simulink model "final"  (R2023b)
settings: Solver=ode4  StartTime=0.0  StopTime=10.0  FixedStep=0.001  RelTol=1e-3
settings Model: Creator=ratho  LastModifiedBy=ratho

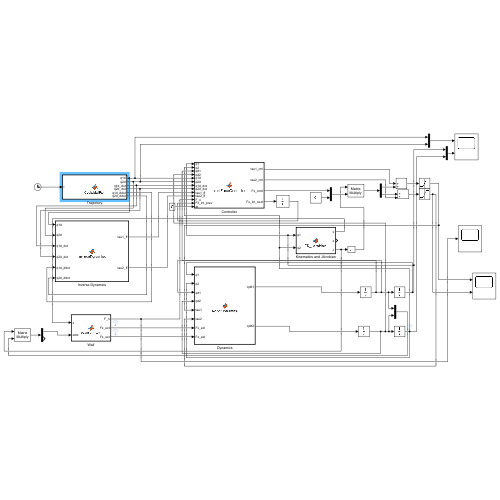
[thumbnail: Simulink's stored preview of the top-level diagram]
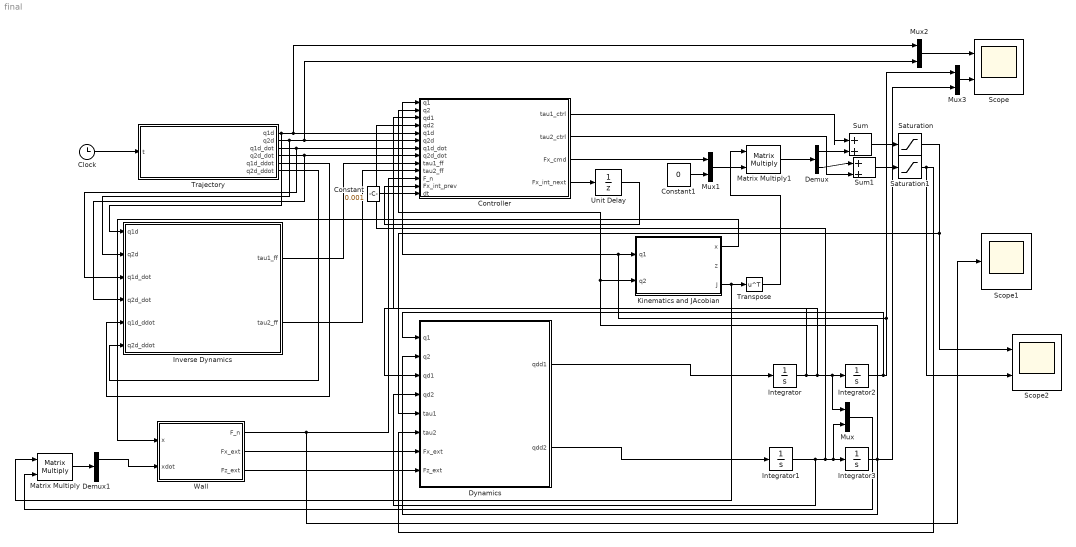
== system final ==
  Clock : Clock
  Constant : Constant  Value=0.001
  Constant1 : Constant  Value=0
  Controller : MATLAB Function  TreatAsAtomicUnit=on
  Demux : Demux  Outputs=2
  Demux1 : Demux  Outputs=2
  Dynamics : MATLAB Function  TreatAsAtomicUnit=on
  Integrator : Integrator
  Integrator1 : Integrator
  Integrator2 : Integrator  InitialCondition=pi/3
  Integrator3 : Integrator  InitialCondition=-pi/4
  Inverse Dynamics : MATLAB Function  TreatAsAtomicUnit=on
  Kinematics and JAcobian : MATLAB Function  TreatAsAtomicUnit=on
  Matrix Multiply : Product  Multiplication=Matrix(*)
  Matrix Multiply1 : Product  Multiplication=Matrix(*)
  Mux{,1..3} (4 alike) : Mux  Inputs=2
  Saturation : Saturate  UpperLimit=400  LowerLimit=-400
  Saturation1 : Saturate  UpperLimit=400  LowerLimit=-400
  Scope : Scope  NumInputPorts=2
  Scope1 : Scope
  Scope2 : Scope  NumInputPorts=2
  Sum : Sum  Inputs=|++
  Sum1 : Sum  Inputs=|++
  Trajectory : MATLAB Function  TreatAsAtomicUnit=on
  Transpose : Math  Operator=transpose
  Unit Delay : UnitDelay  SampleTime=0.001  HasFrameUpgradeWarning=on
  Wall : MATLAB Function  TreatAsAtomicUnit=on
  wires:
  Clock/1 -> Trajectory/1(t)
  Dynamics/1(qdd1) -> Integrator/1
  Dynamics/2(qdd2) -> Integrator1/1
  Integrator/1 -> Dynamics/3(qd1), Controller/3(qd1), Mux/1, Integrator2/1
  Integrator1/1 -> Dynamics/4(qd2), Controller/4(qd2), Mux/2, Integrator3/1
  Integrator2/1 -> Dynamics/1(q1), Mux3/1, Kinematics and JAcobian/1(q1), Controller/1(q1)
  Integrator3/1 -> Mux3/2, Controller/2(q2), Kinematics and JAcobian/2(q2), Dynamics/2(q2)
  Trajectory/1(q1d) -> Mux2/1, Controller/5(q1d), Inverse Dynamics/1(q1d)
  Trajectory/2(q2d) -> Mux2/2, Controller/6(q2d), Inverse Dynamics/2(q2d)
  Trajectory/3(q1d_dot) -> Controller/7(q1d_dot), Inverse Dynamics/3(q1d_dot)
  Trajectory/4(q2d_dot) -> Controller/8(q2d_dot), Inverse Dynamics/4(q2d_dot)
  Trajectory/5(q1d_ddot) -> Inverse Dynamics/5(q1d_ddot)
  Trajectory/6(q2d_ddot) -> Inverse Dynamics/6(q2d_ddot)
  Inverse Dynamics/1(tau1_ff) -> Controller/9(tau1_ff)
  Inverse Dynamics/2(tau2_ff) -> Controller/10(tau2_ff)
  Wall/2(Fx_ext) -> Dynamics/7(Fx_ext)
  Wall/3(Fz_ext) -> Dynamics/8(Fz_ext)
  Kinematics and JAcobian/1(x) -> Wall/1(x)
  Constant/1 -> Controller/13(dt)
  Controller/4(Fx_int_next) -> Unit Delay/1
  Unit Delay/1 -> Controller/12(Fx_int_prev)
  Kinematics and JAcobian/3(J) -> Matrix Multiply/1, Transpose/1
  Mux/1 -> Matrix Multiply/2
  Controller/3(Fx_cmd) -> Mux1/1
  Constant1/1 -> Mux1/2
  Mux1/1 -> Matrix Multiply1/2
  Transpose/1 -> Matrix Multiply1/1
  Matrix Multiply1/1 -> Demux/1
  Demux/2 -> Sum1/1
  Demux/1 -> Sum/2
  Controller/1(tau1_ctrl) -> Sum/1
  Controller/2(tau2_ctrl) -> Sum1/2
  Sum/1 -> Saturation/1
  Sum1/1 -> Saturation1/1
  Matrix Multiply/1 -> Demux1/1
  Demux1/1 -> Wall/2(xdot)
  Saturation/1 -> Scope2/1, Dynamics/5(tau1)
  Saturation1/1 -> Scope2/2, Dynamics/6(tau2)
  Mux2/1 -> Scope/1
  Mux3/1 -> Scope/2
  Wall/1(F_n) -> Scope1/1, Controller/11(F_n)

== matlab function final/Inverse Dynamics ==
  data: q1d input; tau1_ff output; q2d input; q1d_dot input; q2d_dot input; q1d_ddot input; q2d_ddot input; tau2_ff output
function [tau1_ff, tau2_ff] = InverseDynamics( ...
    q1d,q2d,q1d_dot,q2d_dot,q1d_ddot,q2d_ddot)
%#codegen

%% ---- CONSTANTS ----
m1 = 1; m2 = 1;
l1 = 1; l2 = 1;
r1 = l1/2; r2 = l2/2;
I1 = (1/12)*m1*l1^2;
I2 = (1/12)*m2*l2^2;
g  = 9.81;

%% ---- Inertia ----
M11 = I1+I2 + m1*r1^2 + m2*(l1^2+r2^2) + 2*m2*l1*r2*cos(q2d);
M12 = I2 + m2*r2^2 + m2*l1*r2*cos(q2d);
M21 = M12;
M22 = I2 + m2*r2^2;
M = [M11 M12; M21 M22];

%% ---- Coriolis ----
h  = -m2*l1*r2*sin(q2d);
C1 = h*(2*q1d_dot*q2d_dot + q2d_dot^2);
C2 = h*(-q1d_dot^2);
C  = [C1; C2];

%% ---- Gravity ----
G1 = (m1*r1 + m2*l1)*g*cos(q1d) + m2*r2*g*cos(q1d+q2d);
G2 = m2*r2*g*cos(q1d+q2d);
G  = [G1; G2];

tau = M*[q1d_ddot; q2d_ddot] + C + G;

tau1_ff = tau(1);
tau2_ff = tau(2);

end

== matlab function final/Wall ==
  data: x input; F_n output; xdot input; Fx_ext output; Fz_ext output
function [F_n, Fx_ext, Fz_ext] = WallContact(x, xdot)
%#codegen

% ==== CONSTANTS ====
wall_x = 1.75;   % wall position
Kc     = 500;    % stiffness
Dc     = 30;     % damping

% ==== PREDEFINE OUTPUTS AS SCALARS ====
F_n    = 0.0;
Fx_ext = 0.0;
Fz_ext = 0.0;

% ==== PENETRATION (robot is left, wall is to the right) ====
penetration = x - wall_x;

if penetration > 0
    % magnitude of contact force (positive when in compression)
    F_n = Kc*penetration + Dc*xdot;
    if F_n < 0
        F_n = 0;   % safety, shouldn’t really happen
    end
else
    F_n = 0.0;
end

% Force ON THE ROBOT in x (wall pushes back towards -x)
Fx_ext = -F_n;
Fz_ext = 0.0;

end

== matlab function final/Kinematics and JAcobian ==
  data: q1 input; x output; q2 input; z output; J output
function [x, z, J] = FK_Jacobian(q1, q2)
%#codegen

%% ---- CONSTANTS ----
l1 = 1;
l2 = 1;

%% ---- Forward kinematics ----
x = l1*cos(q1) + l2*cos(q1 + q2);
z = l1*sin(q1) + l2*sin(q1 + q2);

%% ---- Jacobian ----
J11 = -l1*sin(q1) - l2*sin(q1 + q2);
J12 = -l2*sin(q1 + q2);
J21 =  l1*cos(q1) + l2*cos(q1 + q2);
J22 =  l2*cos(q1 + q2);
J = [J11 J12; J21 J22];

end

== matlab function final/Controller ==
  data: tau1_ctrl output; tau2_ctrl output; q1 input; Fx_cmd output; q2 input; qd1 input; qd2 input; q1d input; q2d input; q1d_dot input; q2d_dot input; tau1_ff input; tau2_ff input; F_n input; Fx_int_prev input; dt input; Fx_int_next output
function [tau1_ctrl, tau2_ctrl, Fx_cmd, Fx_int_next] = ...
    JointForceController( ...
       q1,q2,qd1,qd2, ...
       q1d,q2d,q1d_dot,q2d_dot, ...
       tau1_ff, tau2_ff, ...
       F_n, Fx_int_prev, dt)
%#codegen

% ==== CONSTANTS ====
% Joint PD gains
Kp1 = 300;   Kd1 = 50;
Kp2 = 300;   Kd2 = 50;

% Force PI gains
Kpf = 30;
Kif = 60;

% Desired NORMAL force magnitude (positive)
F_des = 20;   % N

% ==== Joint-space PD tracking (always active) ====
e1    = q1d - q1;
e2    = q2d - q2;
ed1   = q1d_dot - qd1;
ed2   = q2d_dot - qd2;

tau1_pd = Kp1*e1 + Kd1*ed1;
tau2_pd = Kp2*e2 + Kd2*ed2;

% ==== Force control (only when in contact) ====
if F_n > 0.1      % small threshold to avoid chattering
    eF = F_des - F_n;
    Fx_int_next = Fx_int_prev + eF * dt;
    Fx_cmd = Kpf*eF + Kif*Fx_int_next;
else
    % no contact → no normal force command
    Fx_cmd      = 0.0;
    Fx_int_next = 0.0;  % reset integral when not touching
end

% ==== Total joint torques excluding force term ====
tau1_ctrl = tau1_ff + tau1_pd;
tau2_ctrl = tau2_ff + tau2_pd;

end

== matlab function final/Dynamics ==
  data: q1 input; qdd1 output; q2 input; qd1 input; qd2 input; tau1 input; tau2 input; Fx_ext input; Fz_ext input; qdd2 output
function [qdd1, qdd2] = RobotDynamics(q1,q2,qd1,qd2,tau1,tau2,Fx_ext,Fz_ext)
%#codegen

%% ---- CONSTANTS ----
m1 = 1; m2 = 1;
l1 = 1; l2 = 1;
r1 = l1/2; r2 = l2/2;
I1 = (1/12)*m1*l1^2;
I2 = (1/12)*m2*l2^2;
g  = 9.81;

%% ---- Prepare vectors ----
q  = [q1; q2];
qd = [qd1; qd2];
tau = [tau1; tau2];

%% ---- Inertia matrix ----
M11 = I1+I2 + m1*r1^2 + m2*(l1^2+r2^2) + 2*m2*l1*r2*cos(q2);
M12 = I2 + m2*r2^2 + m2*l1*r2*cos(q2);
M21 = M12;
M22 = I2 + m2*r2^2;
M = [M11 M12; M21 M22];

%% ---- Coriolis ----
h  = -m2*l1*r2*sin(q2);
C1 = h*(2*qd1*qd2 + qd2^2);
C2 = h*(-qd1^2);
C  = [C1; C2];

%% ---- Gravity ----
G1 = (m1*r1 + m2*l1)*g*cos(q1) + m2*r2*g*cos(q1+q2);
G2 = m2*r2*g*cos(q1+q2);
G  = [G1; G2];

%% ---- Jacobian for external force ----
J11 = -l1*sin(q1) - l2*sin(q1 + q2);
J12 = -l2*sin(q1 + q2);
J21 =  l1*cos(q1) + l2*cos(q1 + q2);
J22 =  l2*cos(q1 + q2);
J = [J11 J12; J21 J22];

F_ext = [Fx_ext; Fz_ext];
tau_ext = J' * F_ext;

%% ---- Forward dynamics ----
qdd = M \ (tau + tau_ext - C - G);

qdd1 = qdd(1);
qdd2 = qdd(2);

end

== matlab function final/Trajectory ==
  data: t input; q1d output; q2d output; q1d_dot output; q2d_dot output; q1d_ddot output; q2d_ddot output
function [q1d, q2d, q1d_dot, q2d_dot, q1d_ddot, q2d_ddot] = CycloidalRef(t)
%#codegen

%% ---- CONSTANTS (INSIDE BLOCK) ----
theta1I = pi/3;     
theta1F = 0;

theta2I = -pi/4;    
theta2F = 0;

timeI = 0;          
timeF = 2;

T = timeF - timeI;
A1 = (theta1F - theta1I) / T;
A2 = (theta2F - theta2I) / T;

%% ---- Clamp time ----
if t < timeI
    t = timeI;
elseif t > timeF
    t = timeF;
end

delT = t - timeI;

%% ---- Cycloidal Joint 1 ----
q1d      = theta1I + A1*(delT - (T/(2*pi))*sin((2*pi/T)*delT));
q1d_dot  = A1*(1 - cos((2*pi/T)*delT));
q1d_ddot = (2*pi*A1/T) * sin((2*pi/T)*delT);

%% ---- Cycloidal Joint 2 ----
q2d      = theta2I + A2*(delT - (T/(2*pi))*sin((2*pi/T)*delT));
q2d_dot  = A2*(1 - cos((2*pi/T)*delT));
q2d_ddot = (2*pi*A2/T) * sin((2*pi/T)*delT);

end
